simulink model "Traction_Control_Testing_5_2_2017_pi"  (R2017a)
settings: Solver=VariableStepAuto  StartTime=0.0  StopTime=10  RelTol=1e-3  EnableMultiTasking=on
PreLoadFcn:
  | load CarSim_FE4.mat
  | load Vehicle_information_test_0118_2017.mat
  | 
  | inertiaDriveShaft = 12;
  | ratioDiff = 2;
  | radiusWheel = 16*2.54/100;
  | massVehicle = 1500;
  | inertiaLateral = 25*(radiusWheel)^2;
  | beta = 15;
  | engineRPM0 = 800;
  | tireStiffness = 200000;
  | tireDamping = 1000;
values from neighbouring files (symbols this model uses):
  alpha = 3600    [Traction_Control_parameter.mat]
  FB_S = 1    [Traction_Control_Matlab_Youla.m]    (also in Traction_Control_Testing_main_3_1_17.m = 0)
  M = 50    [Traction_Control_parameter.mat]
  r = 0.26    [Traction_Control_parameter.mat]
  R = 2376    [Traction_Control_parameter.mat]
  Slip_r = 0.2    [Traction_Control_Testing_main_3_1_17.m]
  T = minreal(1-S)    [MAE298_Final_Q2.m]    (also in MAE298_Final_Q22.m = 1-S; MAE298_Final_Q5.m = zpk(minreal(Y*Gp)); MAE_s72A_HW4_Q4.m = 1-S; MAE_s72A_HW4_Q4_5.m = 1-S)
  TR = 4.6    [Traction_Control_parameter.mat]
undefined symbols (not defined in the file or in its folder): sample_time, sigbuilder_block
libraries: fl_lib x27, nesl_utility x18, sdl_lib x8, simulink x2
settings Model: Creator=Ping  LastModifiedBy=Ping
settings OptimizationCC: LifeSpan=inf
settings DebuggingCC: SFUnexpectedBacktrackingDiag=warning  SFNoUnconditionalDefaultTransitionDiag=warning  SFExecutionAtInitializationDiag=none
settings GRTTargetCC: TargetLangStandard=C89/C90 (ANSI)  GeneratePreprocessorConditionals=Disable all
settings ConfigComp: CovMetricSettings=dw  CovHtmlReporting=on  CovSaveCumulativeToWorkspaceVar=on  CovSaveSingleToWorkspaceVar=on  CovExternalEMLEnable=off

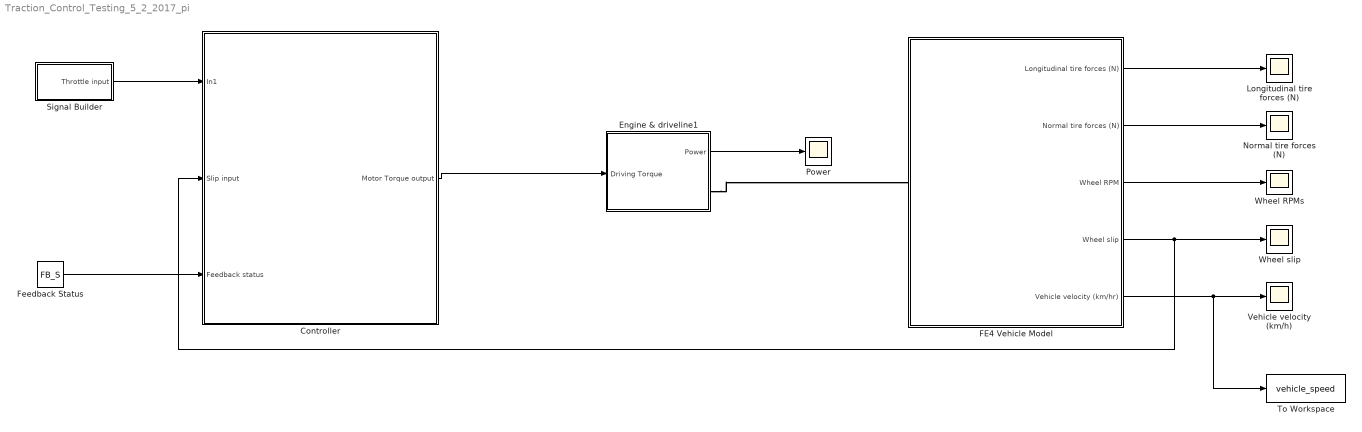
== system Traction_Control_Testing_5_2_2017_pi ==
  Controller : Subsystem
  Engine & driveline1 : Subsystem
  FE4 Vehicle Model : Subsystem
  Feedback Status : Constant  Value=FB_S
  Longitudinal tire forces (N) : Scope
  Normal tire forces (N) : Scope
  Power : Scope
  Signal Builder : Subsystem  Tag=STV Subsys  LoadFcn=sigbuilder_block('load');  StartFcn=sigbuilder_block('start');  StopFcn=sigbuilder_block('stop');  ClipboardFcn=sigbuilder_block('clipboard');  mask(Sigbuilder block){tuvar=[0:10]}
      mask help: Simulink:masks:SigbuilderBlock_MD
      mask init:
      | if ~strcmp(get_param(bdroot(gcbh),'SimulationStatus'),'stopped') tuvar = sigbuilder_block('maskInit'); end
      settings: CopyFcn=sigbuilder_block('copy');  DeleteFcn=sigbuilder_block('delete');  ModelCloseFcn=sigbuilder_block('modelClose');  PreSaveFcn=sigbuilder_block('preSave');  PauseFcn=sigbuilder_block('pause');  ContinueFcn=sigbuilder_block('continue');  NameChangeFcn=sigbuilder_block('namechange');  OpenFcn=sigbuilder_block('open',[118.5 71 550.5 362.5 ]);  CloseFcn=sigbuilder_block('close');
      mask Display: plot(0, 0, 100, 100,[2, 2, 32, 32, 2], [68, 8, 8, 68, 68],[32, 2], [38, 38], [32, 19, 2],[53, 60, 44], [32, 17, 17, 2],[16, 16, 31, 31]);txt = getActiveGroup(gcbh);text(2, 100, txt,'verticalAlignment', 'top');
  To Workspace : ToWorkspace  VariableName=vehicle_speed  SaveFormat=Timeseries  SampleTime=-1
  Vehicle velocity (km/h) : Scope
  Wheel RPMs : Scope
  Wheel slip : Scope
  wires:
  FE4 Vehicle Model/4(Wheel slip) -> Controller/2(Slip input), Wheel slip/1
  FE4 Vehicle Model/2(Normal tire forces (N)) -> Normal tire forces (N)/1
  FE4 Vehicle Model/3(Wheel RPM) -> Wheel RPMs/1
  FE4 Vehicle Model/1(Longitudinal tire forces (N)) -> Longitudinal tire forces (N)/1
  FE4 Vehicle Model/5(Vehicle velocity (km/hr)) -> To Workspace/1, Vehicle velocity (km/h)/1
  Controller/1(Motor Torque output) -> Engine & driveline1/1(Driving Torque)
  Engine & driveline1/1(Power) -> Power/1
  Signal Builder/1(Throttle input) -> Controller/1(In1)
  Feedback Status/1 -> Controller/3(Feedback status)
  connections:
  Engine & driveline1/RConn1 -- FE4 Vehicle Model/LConn1

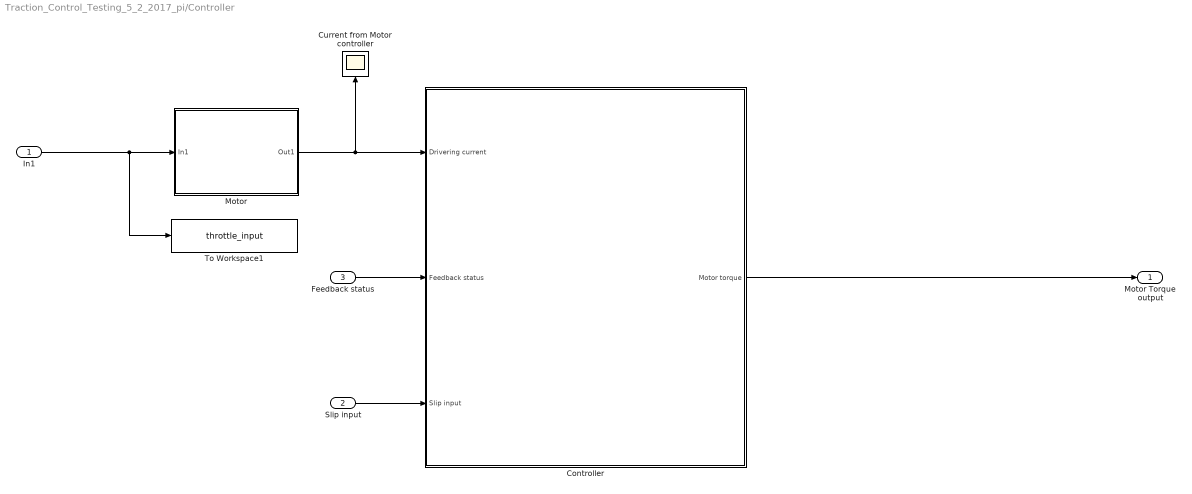
== system Traction_Control_Testing_5_2_2017_pi/Controller ==
  In1 : Inport
  Slip input : Inport  Port=2
  Feedback status : Inport  Port=3
  Controller : Subsystem
  Current from Motor controller : Scope
  Motor : Subsystem
  To Workspace1 : ToWorkspace  VariableName=throttle_input  SaveFormat=Timeseries  SampleTime=-1
  Motor Torque output : Outport
  wires:
  In1/1 -> To Workspace1/1, Motor/1(In1)
  Controller/1(Motor torque) -> Motor Torque output/1
  Motor/1(Out1) -> Current from Motor controller/1, Controller/1(Drivering current)
  Feedback status/1 -> Controller/2(Feedback status)
  Slip input/1 -> Controller/3(Slip input)

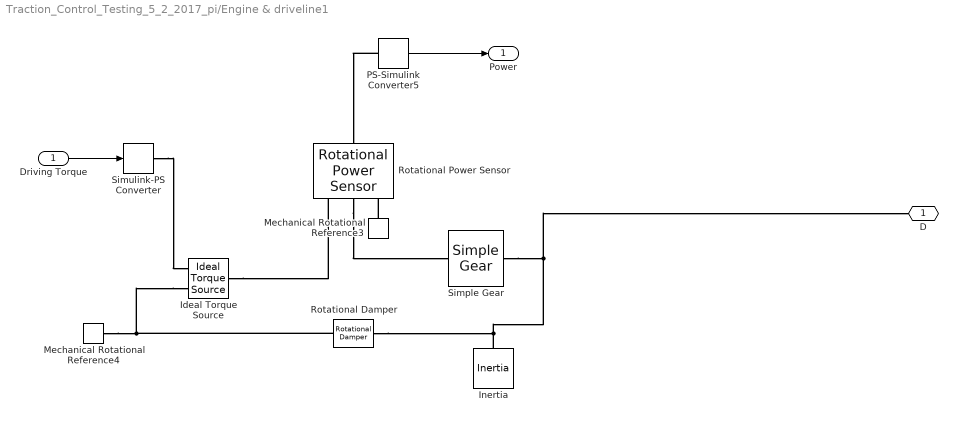
== system Traction_Control_Testing_5_2_2017_pi/Engine & driveline1 ==
  Driving Torque : Inport
  Ideal Torque Source : fl_lib/Mechanical/Mechanical Sources/Ideal Torque Source
  Inertia : fl_lib/Mechanical/Rotational Elements/Inertia  inertia=0.015 kg*m^2  w_specify=on  w_priority=Low  w=0 rad/s  w_nominal_specify=off  w_nominal_unit=rad/s  w_nominal_value=1  t_specify=off  t_priority=Low  t=0 N*m  t_nominal_specify=off  t_nominal_unit=N*m  t_nominal_value=1
  Mechanical Rotational Reference3 : fl_lib/Mechanical/Rotational Elements/Mechanical Rotational Reference
  Mechanical Rotational Reference4 : fl_lib/Mechanical/Rotational Elements/Mechanical Rotational Reference
  PS-Simulink Converter5 : nesl_utility/PS-Simulink Converter  PhysicalDomain=network_engine_domain  SubClassName=ps_output  LeftPortType=input  RightPortType=output  PseudoPeriodic=off  Frequencies=[]  Unit=kW  AffineConversion=off
  Rotational Damper : fl_lib/Mechanical/Rotational Elements/Rotational Damper  D=0.001 N*m/(rad/s)  w_specify=off  w_priority=None  w=0 rad/s  w_nominal_specify=off  w_nominal_unit=rad/s  w_nominal_value=1  t_specify=on  t_priority=Low  t=0 N*m  t_nominal_specify=off  t_nominal_unit=N*m  t_nominal_value=1
  Rotational Power Sensor : sdl_lib/Sensors/Rotational Power Sensor  measurement_type=1  averaging_period=1 s  max_frequency=1000 Hz  max_speed=1000 rpm
      settings: SourceProductName=Simscape Driveline  SourceProductBaseCode=LD
  Simple Gear : sdl_lib/Gears/Simple Gear  ratio=4.6  rotation_direction=1  friction_model=1  T_noload=0.1 N*m  T_nom=5 N*m  efficiency_nom=0.8  efficiency=0.8  mu_visc=[ 0 0 ] N*m/(rad/s)  w_thr=0.01 rad/s  pwr_thr=0.001 W  temperature_TLU=[ 280 300 320 ] K  load_TLU=[ 1 5 10 ] N*m  efficiency_TLU=[ 0.95 0.9 0.85 ]  efficiency_TLU2=[ 0.85 0.8 0.75; 0.95 0.9 0.85; 0.85 0.8 0.7 ]  thermal_mass=50 J/K  T_init=300 K
      settings: SourceProductName=Simscape Driveline
  Simulink-PS Converter : nesl_utility/Simulink-PS Converter  PhysicalDomain=network_engine_domain  SubClassName=ps_input  LeftPortType=input  RightPortType=output  PseudoPeriodic=off  Frequencies=[]  NoiseDistribution=none  NoiseParameters=[]  Unit=N*m  AffineConversion=off  FilteringAndDerivatives=zero  SimscapeFilterOrder=1  InputFilterTimeConstant=0.001  UdotUserProvided=1
  D : PMIOPort  Port=1  Side=Right
  Power : Outport
  wires:
  Driving Torque/1 -> Simulink-PS Converter/1
  PS-Simulink Converter5/1 -> Power/1
  connections:
  Simple Gear/RConn1 -- D/RConn1 -- Rotational Damper/RConn1 -- Inertia/LConn1
  Ideal Torque Source/RConn2 -- Mechanical Rotational Reference4/LConn1 -- Rotational Damper/LConn1
  PS-Simulink Converter5/LConn1 -- Rotational Power Sensor/RConn1
  Mechanical Rotational Reference3/LConn1 -- Rotational Power Sensor/LConn3
  Rotational Power Sensor/LConn2 -- Simple Gear/LConn1
  Simulink-PS Converter/RConn1 -- Ideal Torque Source/RConn1
  Ideal Torque Source/LConn1 -- Rotational Power Sensor/LConn1

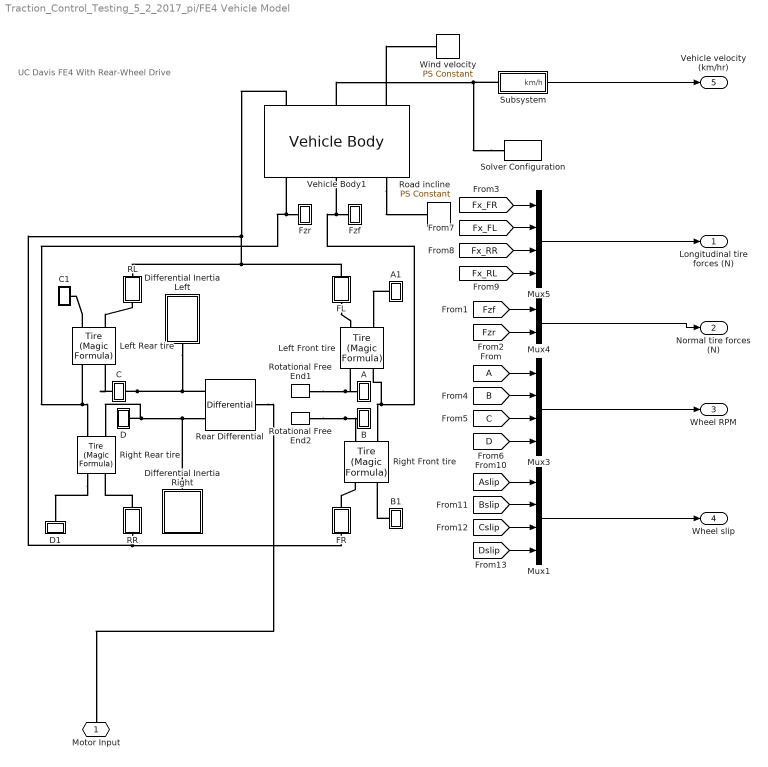
== system Traction_Control_Testing_5_2_2017_pi/FE4 Vehicle Model ==
  note: UC Davis FE4 With Rear-Wheel Drive
  A : Subsystem
  A1 : Subsystem
  B : Subsystem
  B1 : Subsystem
  C : Subsystem
  C1 : Subsystem
  D : Subsystem
  D1 : Subsystem
  Differential Inertia Left : Subsystem
  Differential Inertia Right : Subsystem
  FL : Subsystem
  FR : Subsystem
  Fzf : Subsystem
  Fzr : Subsystem
  Left Front tire : sdl_lib/Tires & Vehicles/Tire (Magic Formula)  parameterization=1  F_z1=3000 N  F_x1=3500 N  kappa1=75  B_m=10  C_m=1.9  D_m=1  E_m=0.97  fz0=4e+3 N  p_Cx=1.685  p_Dx=[ 1.21 -0.037 ]  p_Ex=[ 0.344 0.095 -0.02 0 ]  p_Kx=[ 21.51 -0.163 0.245 ]  p_Hx=[ -0.002 0.002 ]  p_Vx=[ 0 0 ]  v_tr_thr=0.1 m/s  r_e=radiusWheel m  model_compliance=1  stiffness=tireStiffness N/m  damping=tireDamping N/(m/s)  model_inertia=1  inertia=inertiaLateral/2 kg*m^2  initial_velocity=0 rpm  model_resistance=1  resistance_model=1  coeff=0.015  p_tire=250e3 Pa  alpha=-0.003  beta=0.97  coeff_a=84e-4  coeff_b=6.2e-4 s/m  coeff_c=1.6e-4 s^2/m^2  v_thr=1e-3 m/s
      settings: SourceProductName=Simscape Driveline
  Left Rear tire : sdl_lib/Tires & Vehicles/Tire (Magic Formula)  parameterization=1  F_z1=3000 N  F_x1=3500 N  kappa1=75  B_m=10  C_m=1.9  D_m=1  E_m=0.97  fz0=4e+3 N  p_Cx=1.685  p_Dx=[ 1.21 -0.037 ]  p_Ex=[ 0.344 0.095 -0.02 0 ]  p_Kx=[ 21.51 -0.163 0.245 ]  p_Hx=[ -0.002 0.002 ]  p_Vx=[ 0 0 ]  v_tr_thr=0.1 m/s  r_e=radiusWheel m  model_compliance=1  stiffness=tireStiffness N/m  damping=tireDamping N/(m/s)  model_inertia=1  inertia=inertiaLateral/2 kg*m^2  initial_velocity=0 rpm  model_resistance=1  resistance_model=1  coeff=0.015  p_tire=250e3 Pa  alpha=-0.003  beta=0.97  coeff_a=84e-4  coeff_b=6.2e-4 s/m  coeff_c=1.6e-4 s^2/m^2  v_thr=1e-3 m/s
      settings: SourceProductName=Simscape Driveline
  Mux1 : Mux
  Mux3 : Mux
  Mux4 : Mux  Inputs=2
  Mux5 : Mux
  RL : Subsystem
  RR : Subsystem
  Rear Differential : sdl_lib/Gears/Differential  driveshaft_location=2  cd_ratio=1  friction_model=1  efficiency=[ 0.85 0.92 ]  mu_visc=[ 0 0 ] N*m/(rad/s)  pwr_thr=[ 0.001 0.001 ] W  carrier_inertia=0 kg*m^2  planet_inertia=0 kg*m^2  temperature_TLU=[ 280 300 320 ] K  efficiency_ss_TLU=[ 0.95 0.9 0.85 ]  efficiency_cd_TLU=[ 0.95 0.9 0.85 ]  thermal_mass=50 J/K  T_init=300 K
      settings: SourceProductName=Simscape Driveline  SourceProductBaseCode=LD
  Right Front tire : sdl_lib/Tires & Vehicles/Tire (Magic Formula)  parameterization=1  F_z1=3000 N  F_x1=3500 N  kappa1=75  B_m=10  C_m=1.9  D_m=1  E_m=0.97  fz0=4e+3 N  p_Cx=1.685  p_Dx=[ 1.21 -0.037 ]  p_Ex=[ 0.344 0.095 -0.02 0 ]  p_Kx=[ 21.51 -0.163 0.245 ]  p_Hx=[ -0.002 0.002 ]  p_Vx=[ 0 0 ]  v_tr_thr=0.1 m/s  r_e=radiusWheel m  model_compliance=1  stiffness=tireStiffness N/m  damping=tireDamping N/(m/s)  model_inertia=1  inertia=inertiaLateral/2 kg*m^2  initial_velocity=0 rpm  model_resistance=1  resistance_model=1  coeff=0.015  p_tire=250e3 Pa  alpha=-0.003  beta=0.97  coeff_a=84e-4  coeff_b=6.2e-4 s/m  coeff_c=1.6e-4 s^2/m^2  v_thr=1e-3 m/s
      settings: SourceProductName=Simscape Driveline
  Right Rear tire : sdl_lib/Tires & Vehicles/Tire (Magic Formula)  parameterization=1  F_z1=3000 N  F_x1=3500 N  kappa1=75  B_m=10  C_m=1.9  D_m=1  E_m=0.97  fz0=4e+3 N  p_Cx=1.685  p_Dx=[ 1.21 -0.037 ]  p_Ex=[ 0.344 0.095 -0.02 0 ]  p_Kx=[ 21.51 -0.163 0.245 ]  p_Hx=[ -0.002 0.002 ]  p_Vx=[ 0 0 ]  v_tr_thr=0.1 m/s  r_e=radiusWheel m  model_compliance=1  stiffness=tireStiffness N/m  damping=tireDamping N/(m/s)  model_inertia=1  inertia=inertiaLateral/2 kg*m^2  initial_velocity=0 rpm  model_resistance=1  resistance_model=1  coeff=0.015  p_tire=250e3 Pa  alpha=-0.003  beta=0.97  coeff_a=84e-4  coeff_b=6.2e-4 s/m  coeff_c=1.6e-4 s^2/m^2  v_thr=1e-3 m/s
      settings: SourceProductName=Simscape Driveline
  Road incline : fl_lib/Physical Signals/Sources/PS Constant  constant=0
  Rotational Free End1 : fl_lib/Mechanical/Rotational Elements/Rotational Free End  w_specify=on  w_priority=Low  w=0 rad/s  w_nominal_specify=off  w_nominal_unit=rad/s  w_nominal_value=1
      settings: SourceProductName=Simscape  SourceProductBaseCode=SS
  Rotational Free End2 : fl_lib/Mechanical/Rotational Elements/Rotational Free End  w_specify=on  w_priority=Low  w=0 rad/s  w_nominal_specify=off  w_nominal_unit=rad/s  w_nominal_value=1
      settings: SourceProductName=Simscape  SourceProductBaseCode=SS
  Solver Configuration : nesl_utility/Solver Configuration  PhysicalDomain=network_engine_domain  SubClassName=solver  LeftPortType=input  RightPortType=generic  Accelerate=off  Tones=[]  Harmonics=[]  SimulateNoise=off  Profile=off  UseLocalSampling=off  EnableSwitchedLinearOptims=on  FrequencyDomain=off  UseCCode=off  RelTol=0.001  AbsTol=1e-06  MinStep=1e-09  ToWorkspace=off  RevertToSquareIcSolve=off  NumHomotopyIterations=100  PhasorMode=off  PhasorModeNumHarmonics=1  OverrideAbsTol=off  DoDC=off  ResidualTolerance=1e-9  UseLocalSolver=off  LocalSolverChoice=NE_BACKWARD_EULER_ADVANCER  LocalSolverSampleTime=0.1  DoFixedCost=off  MaxNonlinIter=3  MaxModeIter=2  LinearAlgebra=Sparse  DelaysMemoryBudget=1024  AutomaticFiltering=on  FilteringTimeConstant=0.001
  Subsystem : Subsystem
  Vehicle Body1 : sdl_lib/Tires & Vehicles/Vehicle Body  mass=m_total kg  n_w=2  x_f=aa m  x_r=bb m  y_c=hf m  area=frontal_area m^2  Cd=Cd  g=9.81 m/s^2  rho=1.18 kg/m^3  v_specify=on  v_priority=High  v=0 m/s  v_nominal_specify=off  v_nominal_unit=m/s  v_nominal_value=1
      settings: SourceProductName=Simscape Driveline
  Wind velocity : fl_lib/Physical Signals/Sources/PS Constant  constant=0
  Motor Input : PMIOPort  Port=1  Side=Left
  Longitudinal tire forces (N) : Outport
  Normal tire forces (N) : Outport  Port=2
  Wheel RPM : Outport  Port=3
  Wheel slip : Outport  Port=4
  Vehicle velocity (km/hr) : Outport  Port=5
  wires:
  Subsystem/1(km/h) -> Vehicle velocity (km/hr)/1
  [A] -> Mux3/1
  [Fx_FL] -> Mux5/2
  [Fx_FR] -> Mux5/1
  [Fx_RR] -> Mux5/3
  [Fx_RL] -> Mux5/4
  [Aslip] -> Mux1/1
  [Dslip] -> Mux1/4
  Mux1/1 -> Wheel slip/1
  [Bslip] -> Mux1/2
  [Fzr] -> Mux4/2
  Mux4/1 -> Normal tire forces (N)/1
  [Cslip] -> Mux1/3
  [C] -> Mux3/3
  [B] -> Mux3/2
  [D] -> Mux3/4
  Mux3/1 -> Wheel RPM/1
  [Fzf] -> Mux4/1
  Mux5/1 -> Longitudinal tire forces (N)/1
  connections:
  Left Rear tire/RConn1 -- C1/LConn1
  RR/LConn1 -- Right Rear tire/RConn2
  Rotational Free End2/LConn1 -- B/LConn1 -- Right Front tire/LConn2
  Rotational Free End1/LConn1 -- A/LConn1 -- Left Front tire/LConn2
  Rear Differential/LConn1 -- Motor Input/RConn1
  B1/LConn1 -- Right Front tire/RConn1
  Vehicle Body1/LConn3 -- Wind velocity/RConn1
  Right Rear tire/RConn1 -- D1/LConn1
  A1/LConn1 -- Left Front tire/RConn1
  RR/RConn1 -- FR/RConn1 -- Vehicle Body1/LConn1 -- FL/RConn1 -- RL/RConn1
  D/LConn1 -- Right Rear tire/LConn2 -- Differential Inertia Right/RConn1 -- Rear Differential/RConn2
  Fzr/LConn1 -- Left Rear tire/LConn1 -- Right Rear tire/LConn1 -- Vehicle Body1/RConn1
  Solver Configuration/RConn1 -- Vehicle Body1/LConn2 -- Subsystem/LConn1
  Fzf/LConn1 -- Left Front tire/LConn1 -- Right Front tire/LConn1 -- Vehicle Body1/RConn2
  Vehicle Body1/RConn3 -- Road incline/RConn1
  Left Rear tire/RConn2 -- RL/LConn1
  FR/LConn1 -- Right Front tire/RConn2
  FL/LConn1 -- Left Front tire/RConn2
  Rear Differential/RConn1 -- Left Rear tire/LConn2 -- C/LConn1 -- Differential Inertia Left/RConn1

== system Traction_Control_Testing_5_2_2017_pi/Signal Builder ==
  Demux : Demux  Tag=STV Demux  Outputs=1
  FromWs : FromWorkspace  Tag=STV FromWs  VariableName=tuvar  SampleTime=0
      SigBuilderData=|
      | common.afterFinalStr = 'Extrapolate'
      | common.sampleTime = 0
      | dataSet.timeRange = [0 20]
      | dataSet.name = 'Group 1'
      | sbobj.Groups.Name = 'Group 1'
      | sbobj.Groups.Signals.Name = 'Throttle input'
      | sbobj.Groups.Signals.XData = [0 4 4 12 12 20]
      | sbobj.Groups.Signals.YData = [0 0 1 1 0 0]
      | sbobj.Groups.TimeRange = [0 20]
  Throttle input : Outport  Tag=STV Outport
  wires:
  Demux/1 -> Throttle input/1
  FromWs/1 -> Demux/1

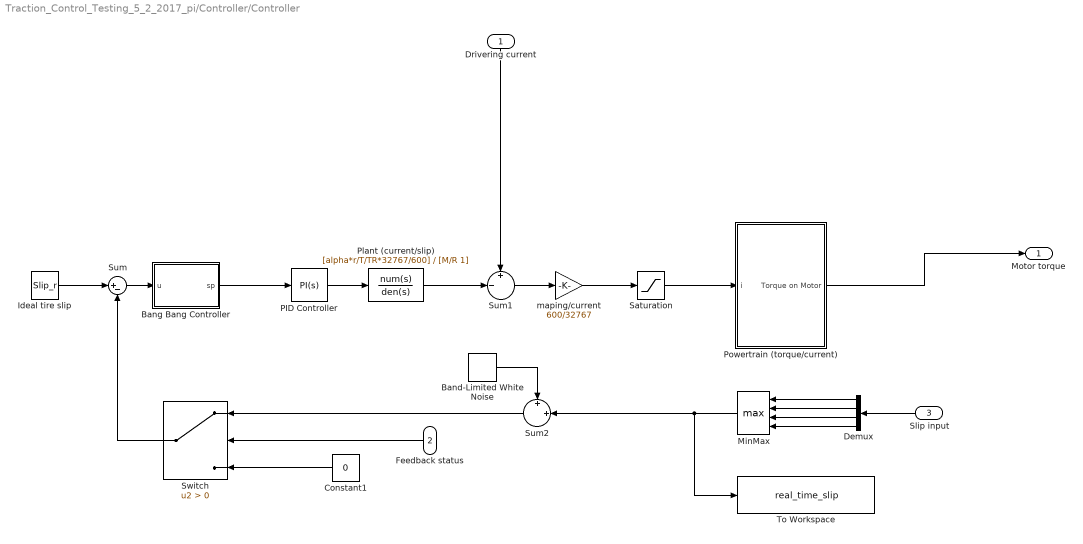
== system Traction_Control_Testing_5_2_2017_pi/Controller/Controller ==
  Drivering current : Inport
  Feedback status : Inport  Port=2
  Slip input : Inport  Port=3
  Band-Limited White Noise : simulink/Sources/Band-Limited White Noise  Cov=power_n  Ts=sample_time  seed=[23341]
  Bang Bang Controller : MATLAB Function  TreatAsAtomicUnit=on
  Constant1 : Constant  Value=0
  Demux : Demux
  Ideal tire slip : Constant  Value=Slip_r
  MinMax : MinMax  Function=max  Inputs=4
  PID Controller : simulink/Continuous/PID Controller  Controller=PI  TimeDomain=Continuous-time  SampleTime=-1  IntegratorMethod=Forward Euler  FilterMethod=Forward Euler  Form=Parallel  UseFilter=on  ControllerParametersSource=internal  P=1  I=1  D=20  N=100  InitialConditionSource=internal  InitialConditionForIntegrator=0  InitialConditionForFilter=0  ExternalReset=none  LimitOutput=off  UpperSaturationLimit=inf  LowerSaturationLimit=-inf  LinearizeAsGain=on  AntiWindupMode=none  Kb=1  TrackingMode=off  Kt=1  PParamMin=[]  PParamMax=[]  IParamMin=[]  IParamMax=[]  DParamMin=[]  DParamMax=[]  NParamMin=[]  NParamMax=[]  KbParamMin=[]  KbParamMax=[]  KtParamMin=[]  KtParamMax=[]  POutMin=[]  POutMax=[]  IOutMin=[]  IOutMax=[]  DOutMin=[]  DOutMax=[]  NOutMin=[]  NOutMax=[]  KbOutMin=[]  KbOutMax=[]  KtOutMin=[]  KtOutMax=[]  IntegratorOutMin=[]  IntegratorOutMax=[]  FilterOutMin=[]  FilterOutMax=[]  SumOutMin=[]  SumOutMax=[]  SumI1OutMin=[]  SumI1OutMax=[]  SumI2OutMin=[]  SumI2OutMax=[]  SumI3OutMin=[]  SumI3OutMax=[]  SumDOutMin=[]  SumDOutMax=[]  SaturationOutMin=[]  SaturationOutMax=[]  IntegratorContinuousStateAttributes=''  IntegratorStateMustResolveToSignalObject=off  IntegratorRTWStateStorageClass=Auto  FilterContinuousStateAttributes=''  FilterStateMustResolveToSignalObject=off  FilterRTWStateStorageClass=Auto  DifferentiatorICPrevScaledInput=0  DifferentiatorOutMin=[]  DifferentiatorOutMax=[]  InitialConditionSetting=State (most efficient)
  Plant (current/slip) : TransferFcn  Numerator=[alpha*r/T/TR*32767/600]  Denominator=[M/R 1]
  Powertrain (torque/current) : Subsystem
  Saturation : Saturate  UpperLimit=600  LowerLimit=0
  Sum : Sum  Inputs=|+-
  Sum1 : Sum  Inputs=+|-||
  Sum2 : Sum  Inputs=+|+||
  Switch : Switch  Criteria=u2 > Threshold
  To Workspace : ToWorkspace  VariableName=real_time_slip  SaveFormat=Timeseries  SampleTime=-1
  maping/current : Gain  Gain=600/32767
  Motor torque : Outport
  wires:
  Plant (current/slip)/1 -> Sum1/2
  Sum/1 -> Bang Bang Controller/1(u)
  Ideal tire slip/1 -> Sum/1
  Drivering current/1 -> Sum1/1
  Switch/1 -> Sum/2
  Constant1/1 -> Switch/3
  Feedback status/1 -> Switch/2
  PID Controller/1 -> Plant (current/slip)/1
  Bang Bang Controller/1(sp) -> PID Controller/1
  Powertrain (torque/current)/1(Torque on Motor) -> Motor torque/1
  MinMax/1 -> To Workspace/1, Sum2/2
  Saturation/1 -> Powertrain (torque/current)/1(i)
  Slip input/1 -> Demux/1
  Demux/1 -> MinMax/1
  Demux/2 -> MinMax/2
  Demux/3 -> MinMax/3
  Demux/4 -> MinMax/4
  Sum1/1 -> maping/current/1
  maping/current/1 -> Saturation/1
  Band-Limited White Noise/1 -> Sum2/1
  Sum2/1 -> Switch/1

== system Traction_Control_Testing_5_2_2017_pi/Controller/Motor ==
  In1 : Inport
  Gain : Gain  Gain=32767
  Out1 : Outport
  wires:
  In1/1 -> Gain/1
  Gain/1 -> Out1/1

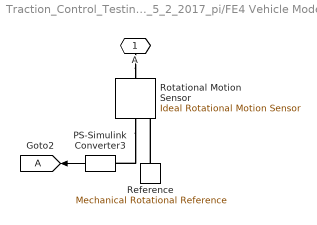
== system Traction_Control_Testing_5_2_2017_pi/FE4 Vehicle Model/A ==
  PS-Simulink Converter3 : nesl_utility/PS-Simulink Converter  PhysicalDomain=network_engine_domain  SubClassName=ps_output  LeftPortType=input  RightPortType=output  PseudoPeriodic=off  Frequencies=[]  Unit=rpm  AffineConversion=off
  Reference : fl_lib/Mechanical/Rotational Elements/Mechanical Rotational Reference
  Rotational Motion Sensor : fl_lib/Mechanical/Mechanical Sensors/Ideal Rotational Motion Sensor  offset=0 rad
  A : PMIOPort  Port=1  Side=Left
  tag scope: A=global
  wires:
  PS-Simulink Converter3/1 -> [A]
  connections:
  Rotational Motion Sensor/RConn2 -- PS-Simulink Converter3/LConn1
  Reference/LConn1 -- Rotational Motion Sensor/RConn1
  A/RConn1 -- Rotational Motion Sensor/LConn1

== system Traction_Control_Testing_5_2_2017_pi/FE4 Vehicle Model/A1 ==
  PS-Simulink Converter : nesl_utility/PS-Simulink Converter  PhysicalDomain=network_engine_domain  SubClassName=ps_output  LeftPortType=input  RightPortType=output  PseudoPeriodic=off  Frequencies=[]  Unit=1  AffineConversion=off
  S : PMIOPort  Port=1  Side=Left
  tag scope: Aslip=global
  wires:
  PS-Simulink Converter/1 -> [Aslip]
  connections:
  S/RConn1 -- PS-Simulink Converter/LConn1

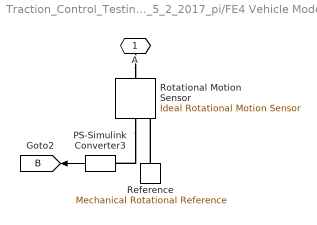
== system Traction_Control_Testing_5_2_2017_pi/FE4 Vehicle Model/B ==
  PS-Simulink Converter3 : nesl_utility/PS-Simulink Converter  PhysicalDomain=network_engine_domain  SubClassName=ps_output  LeftPortType=input  RightPortType=output  PseudoPeriodic=off  Frequencies=[]  Unit=rpm  AffineConversion=off
  Reference : fl_lib/Mechanical/Rotational Elements/Mechanical Rotational Reference
  Rotational Motion Sensor : fl_lib/Mechanical/Mechanical Sensors/Ideal Rotational Motion Sensor  offset=0 rad
  A : PMIOPort  Port=1  Side=Left
  tag scope: B=global
  wires:
  PS-Simulink Converter3/1 -> [B]
  connections:
  A/RConn1 -- Rotational Motion Sensor/LConn1
  Reference/LConn1 -- Rotational Motion Sensor/RConn1
  Rotational Motion Sensor/RConn2 -- PS-Simulink Converter3/LConn1

== system Traction_Control_Testing_5_2_2017_pi/FE4 Vehicle Model/B1 ==
  PS-Simulink Converter : nesl_utility/PS-Simulink Converter  PhysicalDomain=network_engine_domain  SubClassName=ps_output  LeftPortType=input  RightPortType=output  PseudoPeriodic=off  Frequencies=[]  Unit=1  AffineConversion=off
  S : PMIOPort  Port=1  Side=Left
  tag scope: Bslip=global
  wires:
  PS-Simulink Converter/1 -> [Bslip]
  connections:
  S/RConn1 -- PS-Simulink Converter/LConn1

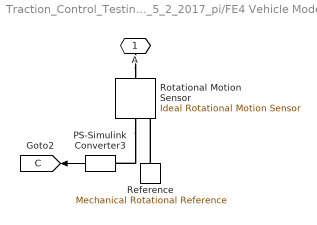
== system Traction_Control_Testing_5_2_2017_pi/FE4 Vehicle Model/C ==
  PS-Simulink Converter3 : nesl_utility/PS-Simulink Converter  PhysicalDomain=network_engine_domain  SubClassName=ps_output  LeftPortType=input  RightPortType=output  PseudoPeriodic=off  Frequencies=[]  Unit=rpm  AffineConversion=off
  Reference : fl_lib/Mechanical/Rotational Elements/Mechanical Rotational Reference
  Rotational Motion Sensor : fl_lib/Mechanical/Mechanical Sensors/Ideal Rotational Motion Sensor  offset=0 rad
  A : PMIOPort  Port=1  Side=Left
  tag scope: C=global
  wires:
  PS-Simulink Converter3/1 -> [C]
  connections:
  Rotational Motion Sensor/RConn2 -- PS-Simulink Converter3/LConn1
  Reference/LConn1 -- Rotational Motion Sensor/RConn1
  A/RConn1 -- Rotational Motion Sensor/LConn1

== system Traction_Control_Testing_5_2_2017_pi/FE4 Vehicle Model/C1 ==
  PS-Simulink Converter : nesl_utility/PS-Simulink Converter  PhysicalDomain=network_engine_domain  SubClassName=ps_output  LeftPortType=input  RightPortType=output  PseudoPeriodic=off  Frequencies=[]  Unit=1  AffineConversion=off
  S : PMIOPort  Port=1  Side=Left
  tag scope: Cslip=global
  wires:
  PS-Simulink Converter/1 -> [Cslip]
  connections:
  S/RConn1 -- PS-Simulink Converter/LConn1

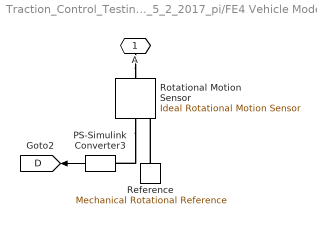
== system Traction_Control_Testing_5_2_2017_pi/FE4 Vehicle Model/D ==
  PS-Simulink Converter3 : nesl_utility/PS-Simulink Converter  PhysicalDomain=network_engine_domain  SubClassName=ps_output  LeftPortType=input  RightPortType=output  PseudoPeriodic=off  Frequencies=[]  Unit=rpm  AffineConversion=off
  Reference : fl_lib/Mechanical/Rotational Elements/Mechanical Rotational Reference
  Rotational Motion Sensor : fl_lib/Mechanical/Mechanical Sensors/Ideal Rotational Motion Sensor  offset=0 rad
  A : PMIOPort  Port=1  Side=Left
  tag scope: D=global
  wires:
  PS-Simulink Converter3/1 -> [D]
  connections:
  A/RConn1 -- Rotational Motion Sensor/LConn1
  Reference/LConn1 -- Rotational Motion Sensor/RConn1
  Rotational Motion Sensor/RConn2 -- PS-Simulink Converter3/LConn1

== system Traction_Control_Testing_5_2_2017_pi/FE4 Vehicle Model/D1 ==
  PS-Simulink Converter : nesl_utility/PS-Simulink Converter  PhysicalDomain=network_engine_domain  SubClassName=ps_output  LeftPortType=input  RightPortType=output  PseudoPeriodic=off  Frequencies=[]  Unit=1  AffineConversion=off
  S : PMIOPort  Port=1  Side=Left
  tag scope: Dslip=global
  wires:
  PS-Simulink Converter/1 -> [Dslip]
  connections:
  S/RConn1 -- PS-Simulink Converter/LConn1

== system Traction_Control_Testing_5_2_2017_pi/FE4 Vehicle Model/Differential Inertia Left ==
  Inertia : fl_lib/Mechanical/Rotational Elements/Inertia  inertia=0.015 kg*m^2  w_specify=on  w_priority=Low  w=0 rad/s  w_nominal_specify=off  w_nominal_unit=rad/s  w_nominal_value=1  t_specify=off  t_priority=Low  t=0 N*m  t_nominal_specify=off  t_nominal_unit=N*m  t_nominal_value=1
  Mechanical Rotational Reference4 : fl_lib/Mechanical/Rotational Elements/Mechanical Rotational Reference
  Rotational Damper : fl_lib/Mechanical/Rotational Elements/Rotational Damper  D=0.001 N*m/(rad/s)  w_specify=off  w_priority=None  w=0 rad/s  w_nominal_specify=off  w_nominal_unit=rad/s  w_nominal_value=1  t_specify=on  t_priority=Low  t=0 N*m  t_nominal_specify=off  t_nominal_unit=N*m  t_nominal_value=1
  Conn1 : PMIOPort  Port=1  Side=Right
  connections:
  Rotational Damper/RConn1 -- Conn1/RConn1 -- Inertia/LConn1
  Rotational Damper/LConn1 -- Mechanical Rotational Reference4/LConn1

== system Traction_Control_Testing_5_2_2017_pi/FE4 Vehicle Model/Differential Inertia Right ==
  Inertia : fl_lib/Mechanical/Rotational Elements/Inertia  inertia=0.015 kg*m^2  w_specify=on  w_priority=Low  w=0 rad/s  w_nominal_specify=off  w_nominal_unit=rad/s  w_nominal_value=1  t_specify=off  t_priority=Low  t=0 N*m  t_nominal_specify=off  t_nominal_unit=N*m  t_nominal_value=1
  Mechanical Rotational Reference4 : fl_lib/Mechanical/Rotational Elements/Mechanical Rotational Reference
  Rotational Damper : fl_lib/Mechanical/Rotational Elements/Rotational Damper  D=0.001 N*m/(rad/s)  w_specify=off  w_priority=None  w=0 rad/s  w_nominal_specify=off  w_nominal_unit=rad/s  w_nominal_value=1  t_specify=on  t_priority=Low  t=0 N*m  t_nominal_specify=off  t_nominal_unit=N*m  t_nominal_value=1
  Conn1 : PMIOPort  Port=1  Side=Right
  connections:
  Rotational Damper/LConn1 -- Mechanical Rotational Reference4/LConn1
  Conn1/RConn1 -- Inertia/LConn1 -- Rotational Damper/RConn1

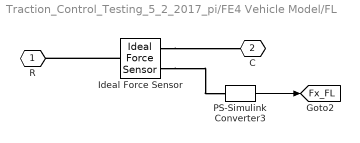
== system Traction_Control_Testing_5_2_2017_pi/FE4 Vehicle Model/FL ==
  Ideal Force Sensor : fl_lib/Mechanical/Mechanical Sensors/Ideal Force Sensor
  PS-Simulink Converter3 : nesl_utility/PS-Simulink Converter  PhysicalDomain=network_engine_domain  SubClassName=ps_output  LeftPortType=input  RightPortType=output  PseudoPeriodic=off  Frequencies=[]  Unit=N  AffineConversion=off
  R : PMIOPort  Port=1  Side=Left
  C : PMIOPort  Port=2  Side=Right
  tag scope: Fx_FL=global
  wires:
  PS-Simulink Converter3/1 -> [Fx_FL]
  connections:
  Ideal Force Sensor/LConn1 -- R/RConn1
  Ideal Force Sensor/RConn1 -- C/RConn1
  Ideal Force Sensor/RConn2 -- PS-Simulink Converter3/LConn1

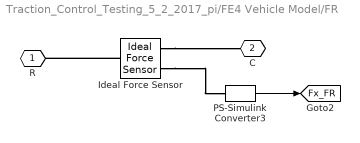
== system Traction_Control_Testing_5_2_2017_pi/FE4 Vehicle Model/FR ==
  Ideal Force Sensor : fl_lib/Mechanical/Mechanical Sensors/Ideal Force Sensor
  PS-Simulink Converter3 : nesl_utility/PS-Simulink Converter  PhysicalDomain=network_engine_domain  SubClassName=ps_output  LeftPortType=input  RightPortType=output  PseudoPeriodic=off  Frequencies=[]  Unit=N  AffineConversion=off
  R : PMIOPort  Port=1  Side=Left
  C : PMIOPort  Port=2  Side=Right
  tag scope: Fx_FR=global
  wires:
  PS-Simulink Converter3/1 -> [Fx_FR]
  connections:
  Ideal Force Sensor/RConn2 -- PS-Simulink Converter3/LConn1
  Ideal Force Sensor/RConn1 -- C/RConn1
  Ideal Force Sensor/LConn1 -- R/RConn1

== system Traction_Control_Testing_5_2_2017_pi/FE4 Vehicle Model/Fzf ==
  PS-Simulink Converter3 : nesl_utility/PS-Simulink Converter  PhysicalDomain=network_engine_domain  SubClassName=ps_output  LeftPortType=input  RightPortType=output  PseudoPeriodic=off  Frequencies=[]  Unit=N  AffineConversion=off
  f : PMIOPort  Port=1  Side=Left
  tag scope: Fzf=global
  wires:
  PS-Simulink Converter3/1 -> [Fzf]
  connections:
  f/RConn1 -- PS-Simulink Converter3/LConn1

== system Traction_Control_Testing_5_2_2017_pi/FE4 Vehicle Model/Fzr ==
  PS-Simulink Converter3 : nesl_utility/PS-Simulink Converter  PhysicalDomain=network_engine_domain  SubClassName=ps_output  LeftPortType=input  RightPortType=output  PseudoPeriodic=off  Frequencies=[]  Unit=N  AffineConversion=off
  f : PMIOPort  Port=1  Side=Left
  tag scope: Fzr=global
  wires:
  PS-Simulink Converter3/1 -> [Fzr]
  connections:
  f/RConn1 -- PS-Simulink Converter3/LConn1

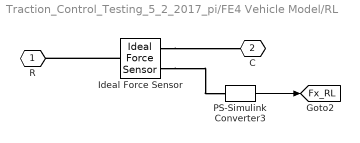
== system Traction_Control_Testing_5_2_2017_pi/FE4 Vehicle Model/RL ==
  Ideal Force Sensor : fl_lib/Mechanical/Mechanical Sensors/Ideal Force Sensor
  PS-Simulink Converter3 : nesl_utility/PS-Simulink Converter  PhysicalDomain=network_engine_domain  SubClassName=ps_output  LeftPortType=input  RightPortType=output  PseudoPeriodic=off  Frequencies=[]  Unit=N  AffineConversion=off
  R : PMIOPort  Port=1  Side=Left
  C : PMIOPort  Port=2  Side=Right
  tag scope: Fx_RL=global
  wires:
  PS-Simulink Converter3/1 -> [Fx_RL]
  connections:
  Ideal Force Sensor/RConn2 -- PS-Simulink Converter3/LConn1
  Ideal Force Sensor/RConn1 -- C/RConn1
  Ideal Force Sensor/LConn1 -- R/RConn1

== system Traction_Control_Testing_5_2_2017_pi/FE4 Vehicle Model/RR ==
  Ideal Force Sensor : fl_lib/Mechanical/Mechanical Sensors/Ideal Force Sensor
  PS-Simulink Converter3 : nesl_utility/PS-Simulink Converter  PhysicalDomain=network_engine_domain  SubClassName=ps_output  LeftPortType=input  RightPortType=output  PseudoPeriodic=off  Frequencies=[]  Unit=N  AffineConversion=off
  R : PMIOPort  Port=1  Side=Left
  C : PMIOPort  Port=2  Side=Right
  tag scope: Fx_RR=global
  wires:
  PS-Simulink Converter3/1 -> [Fx_RR]
  connections:
  Ideal Force Sensor/LConn1 -- R/RConn1
  Ideal Force Sensor/RConn1 -- C/RConn1
  Ideal Force Sensor/RConn2 -- PS-Simulink Converter3/LConn1

== system Traction_Control_Testing_5_2_2017_pi/FE4 Vehicle Model/Subsystem ==
  PS-Simulink Converter1 : nesl_utility/PS-Simulink Converter  PhysicalDomain=network_engine_domain  SubClassName=ps_output  LeftPortType=input  RightPortType=output  PseudoPeriodic=off  Frequencies=[]  Unit=m/s  AffineConversion=off
  m/s2km/h : Gain  Gain=60*60/1000
  V : PMIOPort  Port=1  Side=Left
  km/h : Outport
  wires:
  PS-Simulink Converter1/1 -> m/s2km/h/1
  m/s2km/h/1 -> km/h/1
  connections:
  V/RConn1 -- PS-Simulink Converter1/LConn1

== system Traction_Control_Testing_5_2_2017_pi/Controller/Controller/Powertrain (torque//current) ==
  i : Inport
  Motor parameter : Gain  Gain=T
  Torque on Motor : Outport
  wires:
  i/1 -> Motor parameter/1
  Motor parameter/1 -> Torque on Motor/1

== matlab function Traction_Control_Testing_5_2_2017_pi/Controller/Controller/Bang Bang Controller ==
  data: u input; sp output
function sp = fcn(u)
%Only active while slip signal is negtive 
if u<0
    u_1 = u;
else 
    u_1 = 0;
end

sp = u_1;
